simulink model "wahadlo_stabil"  (R2021b)
settings: Solver=ode1  StartTime=0.0  StopTime=500  FixedStep=1e-3  MaxStep=0.01  MinStep=1e-6  RelTol=1e-2
values from neighbouring files (symbols this model uses):
  n = i    [LAB05_EX1_2.m]    (also in LAB05_EX3.m = 1)
undefined symbols (not defined in the file or in its folder): FullStateFeedbackController
settings Model: Creator=Student  LastModifiedBy=adria
settings SolverCC: InitialStep=0.01  MaxOrder=3  AlgebraicLoopSolver=TrustRegion
settings DataIOCC: SaveFormat=Array  SignalLoggingSaveFormat=ModelDataLogs  SaveOutput=off  SaveTime=off  ReturnWorkspaceOutputs=off  SignalLoggingName=sigsOut
settings OptimizationCC: BlockReduction=off  BooleanDataType=off  ExpressionDepthLimit=2147483647  InitFltsAndDblsToZero=on  LifeSpan=inf
settings DebuggingCC: SaveWithParameterizedLinksMsg=none  UnderspecifiedInitializationDetection=Classic  MergeDetectMultiDrivingBlocksExec=none  SignalResolutionControl=TryResolveAllWithWarning  MultiTaskDSMMsg=warning  MultiTaskCondExecSysMsg=none  FcnCallInpInsideContextMsg=warning  StateNameClashWarn=warning  SFUnexpectedBacktrackingDiag=warning  SFNoUnconditionalDefaultTransitionDiag=warning  SFExecutionAtInitializationDiag=none  SFMachineParentedDataDiag=warning  ArithmeticOperatorsInVariantConditions=warning
settings HardwareCC: ProdBitPerPointer=32  ProdBitPerSizeT=32  ProdBitPerPtrDiffT=32  ProdLargestAtomicFloat=None  ProdIntDivRoundTo=Undefined  ProdEndianess=Unspecified  ProdWordSize=32  ProdHWDeviceType=32-bit Generic  TargetUnknown=on
settings ModelReferenceCC: PropagateSignalLabelsOutOfModel=off
settings SFSimCC: SimUseLocalCustomCode=off  CustomCodeUndefinedFunction=UseInterfaceOnly
settings RTWCC: RTWUseLocalCustomCode=off
settings CodeAppCC: StateflowObjectComments=on
settings GRTTargetCC: TargetFcnLib=ansi_tfl_tmw.mat  TargetLangStandard=C89/C90 (ANSI)  ModelReferenceCompliant=off  ParMdlRefBuildCompliant=off  CompOptLevelCompliant=off  ConcurrentExecutionCompliant=off  CombineOutputUpdateFcns=off  MatFileLogging=off  MATLABClassNameForMDSCustomization=Simulink.SoftwareTarget.TargetSpecificTriggerConfigurationBase  GRTInterface=on
settings ConfigComp: CovMetricSettings=dw  CovSaveCumulativeToWorkspaceVar=on  CovSaveSingleToWorkspaceVar=on  CovExternalEMLEnable=off

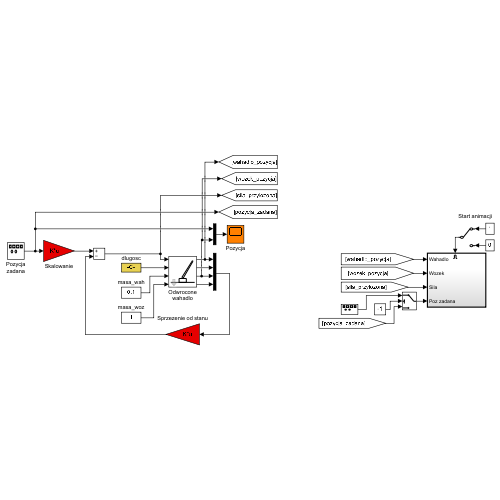
[thumbnail: Simulink's stored preview of the top-level diagram]
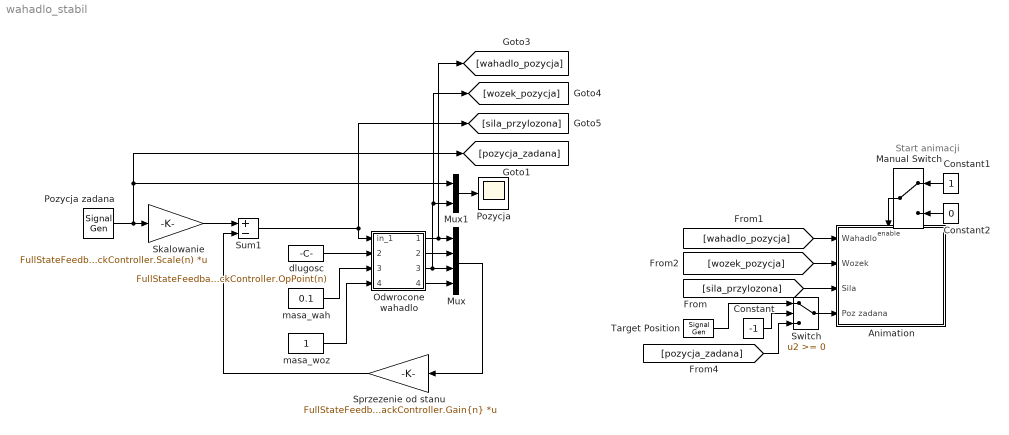
== system wahadlo_stabil ==
  note: Start animacji
  Animation : Subsystem  TreatAsAtomicUnit=on
  Constant : Constant  Value=-1
  Constant1 : Constant
  Constant2 : Constant  Value=0
  Manual Switch : ManualSwitch
  Mux : Mux
  Mux1 : Mux  Inputs=2
  Odwrocone wahadlo : Subsystem  mask(Odwrocone wahadlo){init_cond=[0.1, 0, 0, 0], specs=[48, 0.1, 1.0, 9.8]}
      mask prompts: init_cond "Poczatkowe(kat, predkosc katowa, pozycja wozka,  predkosc wozka):"; specs "Parametry (dlugosc, masa wahadla, masa wozka, g):"
      mask help: Odwrocone wahadlo
      mask init:
      | l=specs(1)/2;m=specs(2);mc=specs(3);g=specs(4);
      mask Help: Odwrocone wahadlo
      mask Display: plot(-4,-1,4,6,[0 3 2.8 -0.2 0],[1 5 5.15 1.15 1],[-1 -1 1 1 -1],[1 0 0 1 1],[-3.5 3.5],[0 0])
  Pozycja : Scope
  Pozycja zadana : SignalGenerator  WaveForm=square  Frequency=0.01
  Skalowanie : Gain  Gain=FullStateFeedbackController.Scale(n)  Multiplication=Matrix(K*u)  SaturateOnIntegerOverflow=on  OutDataTypeStr=Inherit: Same as input  ParamDataTypeStr=Inherit: Same as input
  Sprzezenie od stanu : Gain  Gain=FullStateFeedbackController.Gain{n}  Multiplication=Matrix(K*u)  SaturateOnIntegerOverflow=on  OutDataTypeStr=Inherit: Same as input  ParamDataTypeStr=Inherit: Same as input
  Sum1 : Sum  Inputs=+-  SaturateOnIntegerOverflow=on
  Switch : Switch  SaturateOnIntegerOverflow=on  InputSameDT=on
  Target Position : SignalGenerator  WaveForm=sawtooth  Amplitude=1.500000  Frequency=0.628320  Units=rad/sec
  dlugosc : Constant  Value=FullStateFeedbackController.OpPoint(n)  VectorParams1D=off
  masa_wah : Constant  Value=0.1
  masa_woz : Constant
  wires:
  Sprzezenie od stanu/1 -> Sum1/2
  Odwrocone wahadlo/1(out_1) -> [wahadlo_pozycja], Mux/1
  Odwrocone wahadlo/4(out_4) -> Mux/4
  Odwrocone wahadlo/2(out_2) -> Mux/2
  dlugosc/1 -> Odwrocone wahadlo/2(dlugosc)
  masa_wah/1 -> Odwrocone wahadlo/3(masa_wah)
  masa_woz/1 -> Odwrocone wahadlo/4(masa_woz)
  Odwrocone wahadlo/3(out_3) -> Mux/3, [wozek_pozycja], Mux1/2
  Mux/1 -> Sprzezenie od stanu/1
  Mux1/1 -> Pozycja/1
  Sum1/1 -> Odwrocone wahadlo/1(in_1), [sila_przylozona]
  Skalowanie/1 -> Sum1/1
  Pozycja zadana/1 -> [pozycja_zadana], Mux1/1, Skalowanie/1
  Manual Switch/1 -> Animation/Enable
  Switch/1 -> Animation/4(Poz zadana)
  [wozek_pozycja] -> Animation/2(Wozek)
  [wahadlo_pozycja] -> Animation/1(Wahadlo)
  Constant2/1 -> Manual Switch/2
  [sila_przylozona] -> Animation/3(Sila)
  Constant1/1 -> Manual Switch/1
  Constant/1 -> Switch/2
  [pozycja_zadana] -> Switch/3
  Target Position/1 -> Switch/1

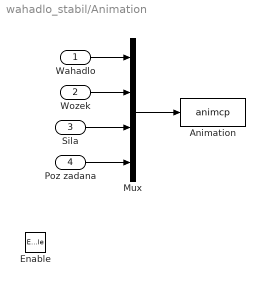
== system wahadlo_stabil/Animation ==
  Wahadlo : Inport
  Wozek : Inport  Port=2
  Sila : Inport  Port=3
  Poz zadana : Inport  Port=4
  Enable : EnablePort
  Animation : S-Function  FunctionName=animcp  SFunctionDeploymentMode=off  EnableBusSupport=off
  Mux : Mux
  wires:
  Mux/1 -> Animation/1
  Wahadlo/1 -> Mux/1
  Sila/1 -> Mux/3
  Poz zadana/1 -> Mux/4
  Wozek/1 -> Mux/2

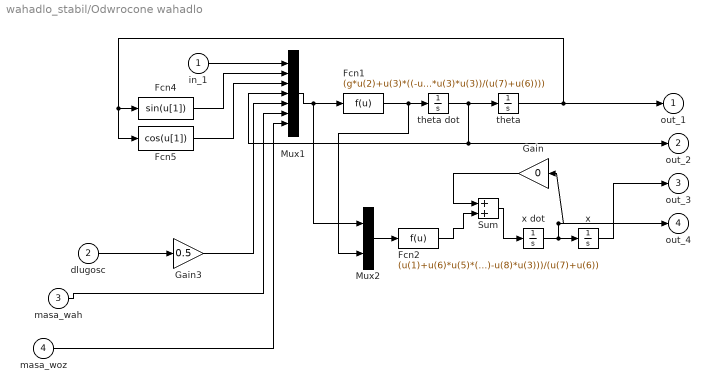
== system wahadlo_stabil/Odwrocone wahadlo ==
  in_1 : Inport
  dlugosc : Inport  Port=2
  masa_wah : Inport  Port=3
  masa_woz : Inport  Port=4
  Fcn1 : Fcn  Expr=(g*u(2)+u(3)*((-u(1)-u(6)*u(5)*u(4)*u(4)*u(2))/(u(7)+u(6))))/(u(5)*(4/3-(u(6)*u(3)*u(3))/(u(7)+u(6))))
  Fcn2 : Fcn  Expr=(u(1)+u(6)*u(5)*(u(4)*u(4)*u(2)-u(8)*u(3)))/(u(7)+u(6))
  Fcn4 : Fcn
  Fcn5 : Fcn  Expr=cos(u[1])
  Gain : Gain  Gain=0  SaturateOnIntegerOverflow=on  OutDataTypeStr=Inherit: Same as input  ParamDataTypeStr=Inherit: Same as input
  Gain3 : Gain  Gain=0.5  SaturateOnIntegerOverflow=on  OutDataTypeStr=Inherit: Same as input  ParamDataTypeStr=Inherit: Same as input
  Mux1 : Mux  Inputs=7
  Mux2 : Mux  Inputs=[7,1]
  Sum : Sum  SaturateOnIntegerOverflow=on
  theta : Integrator  InitialCondition=init_cond(1)
  theta dot : Integrator  InitialCondition=init_cond(2)
  x : Integrator  InitialCondition=init_cond(3)
  x dot : Integrator  InitialCondition=init_cond(4)
  out_1 : Outport  InitialOutput=0  VectorParamsAs1DForOutWhenUnconnected=off
  out_2 : Outport  Port=2  InitialOutput=0  VectorParamsAs1DForOutWhenUnconnected=off
  out_3 : Outport  Port=3  InitialOutput=0  VectorParamsAs1DForOutWhenUnconnected=off
  out_4 : Outport  Port=4  InitialOutput=0  VectorParamsAs1DForOutWhenUnconnected=off
  wires:
  in_1/1 -> Mux1/1
  x/1 -> out_3/1
  x dot/1 -> x/1, out_4/1, Gain/1
  Mux1/1 -> Fcn1/1, Mux2/1
  Mux2/1 -> Fcn2/1
  Fcn1/1 -> theta dot/1, Mux2/2
  theta dot/1 -> Mux1/4, out_2/1, theta/1
  Fcn4/1 -> Mux1/2
  Fcn5/1 -> Mux1/3
  theta/1 -> out_1/1, Fcn4/1, Fcn5/1
  Sum/1 -> x dot/1
  Fcn2/1 -> Sum/2
  Gain/1 -> Sum/1
  dlugosc/1 -> Gain3/1
  masa_wah/1 -> Mux1/6
  masa_woz/1 -> Mux1/7
  Gain3/1 -> Mux1/5
